simulink model "AariaJoystickR2017a"  (R2017a)
settings: Solver=VariableStepAuto  StartTime=0.0  StopTime=inf  FixedStep=0.1  RelTol=1e-3  EnableMultiTasking=on
model workspace (MATLAB code in the model file):
  | my_a =1;
undefined symbols (not defined in the file or in its folder): AARIAENV, AARIAMAN, AARIASEN, Camera, sensor, Source_TS, X, Y, Z
libraries: sm_lib x723, nesl_utility x640, dspmathops x314, simulink x168, vrlib x2, powerlib_meascontrol x1, aerolibanimutils x1, aerolibutil x1
(part 13 of 26)

== system AariaJoystickR2017a/Tool Sensors/Tool sensor2/placeholder noise2 ==
  Constant : Constant  Value=[1 1 1; 1 1 1; 1 1 1]
  Product : Product
  Uniform Random Number : UniformRandomNumber  Minimum=-0.01  Maximum=0.01  SampleTime=0.1
  noise : Outport
  wires:
  Constant/1 -> Product/1
  Product/1 -> noise/1
  Uniform Random Number/1 -> Product/2

== system AariaJoystickR2017a/Base/BaseVSS/BaseEmpty/IMU Base ==
  Sensor Module1 : Subsystem  mask{nL=nL, nS=1}
      mask prompts: nL "Link Number"; nS "Sensor ID of that link"
      mask DialogControl DescGroupVar Prompt: Virtual IMU
      mask DialogControl DescTextVar Prompt: Measures Connected Body's acceleration and angular velocity in the given point
      mask DialogControl Control2 Prompt: The following numbers defines the corresponding numbers for this sensor to read from the parameters file
  Body Coord : PMIOPort  Port=1  Side=Left
  Reference Coord : PMIOPort  Port=2  Side=Left
  Out1 : Outport
  Out2 : Outport  Port=2
  Out3 : Outport  Port=3
  Out4 : Outport  Port=4
  wires:
  Sensor Module1/3(Out2) -> Out3/1
  Sensor Module1/2(Out4) -> Out2/1
  Sensor Module1/4(Out3) -> Out4/1
  Sensor Module1/1(Out5) -> Out1/1
  connections:
  Sensor Module1/LConn2 -- Reference Coord/RConn1
  Sensor Module1/LConn1 -- Body Coord/RConn1

== system AariaJoystickR2017a/Base/BaseVSS/BaseMotion/IMU Base ==
  Sensor Module1 : Subsystem  mask{nL=nL, nS=1}
      mask prompts: nL "Link Number"; nS "Sensor ID of that link"
      mask DialogControl DescGroupVar Prompt: Virtual IMU
      mask DialogControl DescTextVar Prompt: Measures Connected Body's acceleration and angular velocity in the given point
      mask DialogControl Control2 Prompt: The following numbers defines the corresponding numbers for this sensor to read from the parameters file
  Body Coord : PMIOPort  Port=1  Side=Left
  Reference Coord : PMIOPort  Port=2  Side=Left
  Out1 : Outport
  Out2 : Outport  Port=2
  Out3 : Outport  Port=3
  Out4 : Outport  Port=4
  wires:
  Sensor Module1/3(Out2) -> Out3/1
  Sensor Module1/2(Out4) -> Out2/1
  Sensor Module1/4(Out3) -> Out4/1
  Sensor Module1/1(Out5) -> Out1/1
  connections:
  Sensor Module1/LConn2 -- Reference Coord/RConn1
  Sensor Module1/LConn1 -- Body Coord/RConn1

== system AariaJoystickR2017a/Base/BaseVSS/BaseMotion/x 2motion2 ==
  X : Inport
  Difference : simulink/Discrete/Difference  ICPrevInput=1  InputProcessing=Inherited  OutMin=[]  OutMax=[]  OutDataType=fixdt(1, 16)  OutScaling=2^-10  DoSatur=off
  Difference1 : simulink/Discrete/Difference  ICPrevInput=0  InputProcessing=Inherited  OutMin=[]  OutMax=[]  OutDataType=fixdt(1, 16)  OutScaling=2^-10  DoSatur=off
  Simulink-PS Converter : nesl_utility/Simulink-PS Converter  PhysicalDomain=network_engine_domain  SubClassName=ps_input  LeftPortType=input  RightPortType=output  PseudoPeriodic=off  Frequencies=[]  NoiseDistribution=none  NoiseParameters=[]  Unit=1  AffineConversion=off  FilteringAndDerivatives=provide  SimscapeFilterOrder=1  InputFilterTimeConstant=0.001  UdotUserProvided=2
  Motion for PS : PMIOPort  Port=1  Side=Right
  wires:
  X/1 -> Simulink-PS Converter/1, Difference1/1
  Difference/1 -> Simulink-PS Converter/3
  Difference1/1 -> Difference/1, Simulink-PS Converter/2
  connections:
  Simulink-PS Converter/RConn1 -- Motion for PS/RConn1

== system AariaJoystickR2017a/Base/BaseVSS/BaseMotion/x 2motion3 ==
  X : Inport
  Difference : simulink/Discrete/Difference  ICPrevInput=1  InputProcessing=Inherited  OutMin=[]  OutMax=[]  OutDataType=fixdt(1, 16)  OutScaling=2^-10  DoSatur=off
  Difference1 : simulink/Discrete/Difference  ICPrevInput=0  InputProcessing=Inherited  OutMin=[]  OutMax=[]  OutDataType=fixdt(1, 16)  OutScaling=2^-10  DoSatur=off
  Simulink-PS Converter : nesl_utility/Simulink-PS Converter  PhysicalDomain=network_engine_domain  SubClassName=ps_input  LeftPortType=input  RightPortType=output  PseudoPeriodic=off  Frequencies=[]  NoiseDistribution=none  NoiseParameters=[]  Unit=1  AffineConversion=off  FilteringAndDerivatives=provide  SimscapeFilterOrder=1  InputFilterTimeConstant=0.001  UdotUserProvided=2
  Motion for PS : PMIOPort  Port=1  Side=Right
  wires:
  Difference1/1 -> Simulink-PS Converter/2, Difference/1
  Difference/1 -> Simulink-PS Converter/3
  X/1 -> Difference1/1, Simulink-PS Converter/1
  connections:
  Simulink-PS Converter/RConn1 -- Motion for PS/RConn1

== system AariaJoystickR2017a/Base/BaseVSS/BaseMotion/x 2motion4 ==
  X : Inport
  Difference : simulink/Discrete/Difference  ICPrevInput=1  InputProcessing=Inherited  OutMin=[]  OutMax=[]  OutDataType=fixdt(1, 16)  OutScaling=2^-10  DoSatur=off
  Difference1 : simulink/Discrete/Difference  ICPrevInput=0  InputProcessing=Inherited  OutMin=[]  OutMax=[]  OutDataType=fixdt(1, 16)  OutScaling=2^-10  DoSatur=off
  Simulink-PS Converter : nesl_utility/Simulink-PS Converter  PhysicalDomain=network_engine_domain  SubClassName=ps_input  LeftPortType=input  RightPortType=output  PseudoPeriodic=off  Frequencies=[]  NoiseDistribution=none  NoiseParameters=[]  Unit=1  AffineConversion=off  FilteringAndDerivatives=provide  SimscapeFilterOrder=1  InputFilterTimeConstant=0.001  UdotUserProvided=2
  Motion for PS : PMIOPort  Port=1  Side=Right
  wires:
  X/1 -> Simulink-PS Converter/1, Difference1/1
  Difference/1 -> Simulink-PS Converter/3
  Difference1/1 -> Difference/1, Simulink-PS Converter/2
  connections:
  Simulink-PS Converter/RConn1 -- Motion for PS/RConn1

== system AariaJoystickR2017a/Base/BaseVSS/BaseMotion/x 2motion5 ==
  X : Inport
  Difference : simulink/Discrete/Difference  ICPrevInput=1  InputProcessing=Inherited  OutMin=[]  OutMax=[]  OutDataType=fixdt(1, 16)  OutScaling=2^-10  DoSatur=off
  Difference1 : simulink/Discrete/Difference  ICPrevInput=0  InputProcessing=Inherited  OutMin=[]  OutMax=[]  OutDataType=fixdt(1, 16)  OutScaling=2^-10  DoSatur=off
  Simulink-PS Converter : nesl_utility/Simulink-PS Converter  PhysicalDomain=network_engine_domain  SubClassName=ps_input  LeftPortType=input  RightPortType=output  PseudoPeriodic=off  Frequencies=[]  NoiseDistribution=none  NoiseParameters=[]  Unit=1  AffineConversion=off  FilteringAndDerivatives=provide  SimscapeFilterOrder=1  InputFilterTimeConstant=0.001  UdotUserProvided=2
  Motion for PS : PMIOPort  Port=1  Side=Right
  wires:
  Difference1/1 -> Simulink-PS Converter/2, Difference/1
  Difference/1 -> Simulink-PS Converter/3
  X/1 -> Difference1/1, Simulink-PS Converter/1
  connections:
  Simulink-PS Converter/RConn1 -- Motion for PS/RConn1

== system AariaJoystickR2017a/Base/BaseVSS/BaseMotion/x 2motion6 ==
  X : Inport
  Difference : simulink/Discrete/Difference  ICPrevInput=1  InputProcessing=Inherited  OutMin=[]  OutMax=[]  OutDataType=fixdt(1, 16)  OutScaling=2^-10  DoSatur=off
  Difference1 : simulink/Discrete/Difference  ICPrevInput=0  InputProcessing=Inherited  OutMin=[]  OutMax=[]  OutDataType=fixdt(1, 16)  OutScaling=2^-10  DoSatur=off
  Simulink-PS Converter : nesl_utility/Simulink-PS Converter  PhysicalDomain=network_engine_domain  SubClassName=ps_input  LeftPortType=input  RightPortType=output  PseudoPeriodic=off  Frequencies=[]  NoiseDistribution=none  NoiseParameters=[]  Unit=1  AffineConversion=off  FilteringAndDerivatives=provide  SimscapeFilterOrder=1  InputFilterTimeConstant=0.001  UdotUserProvided=2
  Motion for PS : PMIOPort  Port=1  Side=Right
  wires:
  X/1 -> Simulink-PS Converter/1, Difference1/1
  Difference/1 -> Simulink-PS Converter/3
  Difference1/1 -> Difference/1, Simulink-PS Converter/2
  connections:
  Simulink-PS Converter/RConn1 -- Motion for PS/RConn1

== system AariaJoystickR2017a/Base/BaseVSS/BaseMotion/x 2motion7 ==
  X : Inport
  Difference : simulink/Discrete/Difference  ICPrevInput=1  InputProcessing=Inherited  OutMin=[]  OutMax=[]  OutDataType=fixdt(1, 16)  OutScaling=2^-10  DoSatur=off
  Difference1 : simulink/Discrete/Difference  ICPrevInput=0  InputProcessing=Inherited  OutMin=[]  OutMax=[]  OutDataType=fixdt(1, 16)  OutScaling=2^-10  DoSatur=off
  Simulink-PS Converter : nesl_utility/Simulink-PS Converter  PhysicalDomain=network_engine_domain  SubClassName=ps_input  LeftPortType=input  RightPortType=output  PseudoPeriodic=off  Frequencies=[]  NoiseDistribution=none  NoiseParameters=[]  Unit=1  AffineConversion=off  FilteringAndDerivatives=provide  SimscapeFilterOrder=1  InputFilterTimeConstant=0.001  UdotUserProvided=2
  Motion for PS : PMIOPort  Port=1  Side=Right
  wires:
  Difference1/1 -> Simulink-PS Converter/2, Difference/1
  Difference/1 -> Simulink-PS Converter/3
  X/1 -> Difference1/1, Simulink-PS Converter/1
  connections:
  Simulink-PS Converter/RConn1 -- Motion for PS/RConn1

== system AariaJoystickR2017a/Base/BaseVSS/BaseTorque/IMU Base ==
  Sensor Module1 : Subsystem  mask{nL=nL, nS=1}
      mask prompts: nL "Link Number"; nS "Sensor ID of that link"
      mask DialogControl DescGroupVar Prompt: Virtual IMU
      mask DialogControl DescTextVar Prompt: Measures Connected Body's acceleration and angular velocity in the given point
      mask DialogControl Control2 Prompt: The following numbers defines the corresponding numbers for this sensor to read from the parameters file
  Body Coord : PMIOPort  Port=1  Side=Left
  Reference Coord : PMIOPort  Port=2  Side=Left
  Out1 : Outport
  Out2 : Outport  Port=2
  Out3 : Outport  Port=3
  Out4 : Outport  Port=4
  wires:
  Sensor Module1/3(Out2) -> Out3/1
  Sensor Module1/2(Out4) -> Out2/1
  Sensor Module1/4(Out3) -> Out4/1
  Sensor Module1/1(Out5) -> Out1/1
  connections:
  Sensor Module1/LConn2 -- Reference Coord/RConn1
  Sensor Module1/LConn1 -- Body Coord/RConn1

== system AariaJoystickR2017a/Base/BaseVSS/BaseTorque/x 2motion2 ==
  X : Inport
  Difference : simulink/Discrete/Difference  ICPrevInput=1  InputProcessing=Inherited  OutMin=[]  OutMax=[]  OutDataType=fixdt(1, 16)  OutScaling=2^-10  DoSatur=off
  Difference1 : simulink/Discrete/Difference  ICPrevInput=0  InputProcessing=Inherited  OutMin=[]  OutMax=[]  OutDataType=fixdt(1, 16)  OutScaling=2^-10  DoSatur=off
  Simulink-PS Converter : nesl_utility/Simulink-PS Converter  PhysicalDomain=network_engine_domain  SubClassName=ps_input  LeftPortType=input  RightPortType=output  PseudoPeriodic=off  Frequencies=[]  NoiseDistribution=none  NoiseParameters=[]  Unit=1  AffineConversion=off  FilteringAndDerivatives=provide  SimscapeFilterOrder=1  InputFilterTimeConstant=0.001  UdotUserProvided=2
  Motion for PS : PMIOPort  Port=1  Side=Right
  wires:
  X/1 -> Simulink-PS Converter/1, Difference1/1
  Difference/1 -> Simulink-PS Converter/3
  Difference1/1 -> Difference/1, Simulink-PS Converter/2
  connections:
  Simulink-PS Converter/RConn1 -- Motion for PS/RConn1

== system AariaJoystickR2017a/Base/BaseVSS/BaseTorque/x 2motion3 ==
  X : Inport
  Difference : simulink/Discrete/Difference  ICPrevInput=1  InputProcessing=Inherited  OutMin=[]  OutMax=[]  OutDataType=fixdt(1, 16)  OutScaling=2^-10  DoSatur=off
  Difference1 : simulink/Discrete/Difference  ICPrevInput=0  InputProcessing=Inherited  OutMin=[]  OutMax=[]  OutDataType=fixdt(1, 16)  OutScaling=2^-10  DoSatur=off
  Simulink-PS Converter : nesl_utility/Simulink-PS Converter  PhysicalDomain=network_engine_domain  SubClassName=ps_input  LeftPortType=input  RightPortType=output  PseudoPeriodic=off  Frequencies=[]  NoiseDistribution=none  NoiseParameters=[]  Unit=1  AffineConversion=off  FilteringAndDerivatives=provide  SimscapeFilterOrder=1  InputFilterTimeConstant=0.001  UdotUserProvided=2
  Motion for PS : PMIOPort  Port=1  Side=Right
  wires:
  Difference1/1 -> Simulink-PS Converter/2, Difference/1
  Difference/1 -> Simulink-PS Converter/3
  X/1 -> Difference1/1, Simulink-PS Converter/1
  connections:
  Simulink-PS Converter/RConn1 -- Motion for PS/RConn1

== system AariaJoystickR2017a/Base/BaseVSS/BaseTorque/x 2motion4 ==
  X : Inport
  Difference : simulink/Discrete/Difference  ICPrevInput=1  InputProcessing=Inherited  OutMin=[]  OutMax=[]  OutDataType=fixdt(1, 16)  OutScaling=2^-10  DoSatur=off
  Difference1 : simulink/Discrete/Difference  ICPrevInput=0  InputProcessing=Inherited  OutMin=[]  OutMax=[]  OutDataType=fixdt(1, 16)  OutScaling=2^-10  DoSatur=off
  Simulink-PS Converter : nesl_utility/Simulink-PS Converter  PhysicalDomain=network_engine_domain  SubClassName=ps_input  LeftPortType=input  RightPortType=output  PseudoPeriodic=off  Frequencies=[]  NoiseDistribution=none  NoiseParameters=[]  Unit=1  AffineConversion=off  FilteringAndDerivatives=provide  SimscapeFilterOrder=1  InputFilterTimeConstant=0.001  UdotUserProvided=2
  Motion for PS : PMIOPort  Port=1  Side=Right
  wires:
  X/1 -> Simulink-PS Converter/1, Difference1/1
  Difference/1 -> Simulink-PS Converter/3
  Difference1/1 -> Difference/1, Simulink-PS Converter/2
  connections:
  Simulink-PS Converter/RConn1 -- Motion for PS/RConn1

== system AariaJoystickR2017a/Base/BaseVSS/BaseTorque/x 2motion5 ==
  X : Inport
  Difference : simulink/Discrete/Difference  ICPrevInput=1  InputProcessing=Inherited  OutMin=[]  OutMax=[]  OutDataType=fixdt(1, 16)  OutScaling=2^-10  DoSatur=off
  Difference1 : simulink/Discrete/Difference  ICPrevInput=0  InputProcessing=Inherited  OutMin=[]  OutMax=[]  OutDataType=fixdt(1, 16)  OutScaling=2^-10  DoSatur=off
  Simulink-PS Converter : nesl_utility/Simulink-PS Converter  PhysicalDomain=network_engine_domain  SubClassName=ps_input  LeftPortType=input  RightPortType=output  PseudoPeriodic=off  Frequencies=[]  NoiseDistribution=none  NoiseParameters=[]  Unit=1  AffineConversion=off  FilteringAndDerivatives=provide  SimscapeFilterOrder=1  InputFilterTimeConstant=0.001  UdotUserProvided=2
  Motion for PS : PMIOPort  Port=1  Side=Right
  wires:
  Difference1/1 -> Simulink-PS Converter/2, Difference/1
  Difference/1 -> Simulink-PS Converter/3
  X/1 -> Difference1/1, Simulink-PS Converter/1
  connections:
  Simulink-PS Converter/RConn1 -- Motion for PS/RConn1

== system AariaJoystickR2017a/Base/BaseVSS/BaseTorque/x 2motion6 ==
  X : Inport
  Difference : simulink/Discrete/Difference  ICPrevInput=1  InputProcessing=Inherited  OutMin=[]  OutMax=[]  OutDataType=fixdt(1, 16)  OutScaling=2^-10  DoSatur=off
  Difference1 : simulink/Discrete/Difference  ICPrevInput=0  InputProcessing=Inherited  OutMin=[]  OutMax=[]  OutDataType=fixdt(1, 16)  OutScaling=2^-10  DoSatur=off
  Simulink-PS Converter : nesl_utility/Simulink-PS Converter  PhysicalDomain=network_engine_domain  SubClassName=ps_input  LeftPortType=input  RightPortType=output  PseudoPeriodic=off  Frequencies=[]  NoiseDistribution=none  NoiseParameters=[]  Unit=1  AffineConversion=off  FilteringAndDerivatives=provide  SimscapeFilterOrder=1  InputFilterTimeConstant=0.001  UdotUserProvided=2
  Motion for PS : PMIOPort  Port=1  Side=Right
  wires:
  X/1 -> Simulink-PS Converter/1, Difference1/1
  Difference/1 -> Simulink-PS Converter/3
  Difference1/1 -> Difference/1, Simulink-PS Converter/2
  connections:
  Simulink-PS Converter/RConn1 -- Motion for PS/RConn1

== system AariaJoystickR2017a/Base/BaseVSS/BaseTorque/x 2motion7 ==
  X : Inport
  Difference : simulink/Discrete/Difference  ICPrevInput=1  InputProcessing=Inherited  OutMin=[]  OutMax=[]  OutDataType=fixdt(1, 16)  OutScaling=2^-10  DoSatur=off
  Difference1 : simulink/Discrete/Difference  ICPrevInput=0  InputProcessing=Inherited  OutMin=[]  OutMax=[]  OutDataType=fixdt(1, 16)  OutScaling=2^-10  DoSatur=off
  Simulink-PS Converter : nesl_utility/Simulink-PS Converter  PhysicalDomain=network_engine_domain  SubClassName=ps_input  LeftPortType=input  RightPortType=output  PseudoPeriodic=off  Frequencies=[]  NoiseDistribution=none  NoiseParameters=[]  Unit=1  AffineConversion=off  FilteringAndDerivatives=provide  SimscapeFilterOrder=1  InputFilterTimeConstant=0.001  UdotUserProvided=2
  Motion for PS : PMIOPort  Port=1  Side=Right
  wires:
  Difference1/1 -> Simulink-PS Converter/2, Difference/1
  Difference/1 -> Simulink-PS Converter/3
  X/1 -> Difference1/1, Simulink-PS Converter/1
  connections:
  Simulink-PS Converter/RConn1 -- Motion for PS/RConn1

== system AariaJoystickR2017a/Joint1/JointVSS/PrismaticMotion/IMU Sensors ==
  Sensor Module1 : Subsystem  mask{nL=nL, nS=1}
      mask prompts: nL "Link Number"; nS "Sensor ID of that link"
      mask DialogControl DescGroupVar Prompt: Virtual IMU
      mask DialogControl DescTextVar Prompt: Measures Connected Body's acceleration and angular velocity in the given point
      mask DialogControl Control2 Prompt: The following numbers defines the corresponding numbers for this sensor to read from the parameters file
  Sensor Module2 : Subsystem  mask{nL=nL, nS=2}
      mask prompts: nL "Link Number"; nS "Sensor ID of that link"
      mask DialogControl DescGroupVar Prompt: Virtual IMU
      mask DialogControl DescTextVar Prompt: Measures Connected Body's acceleration and angular velocity in the given point
      mask DialogControl Control2 Prompt: The following numbers defines the corresponding numbers for this sensor to read from the parameters file
  Terminator{,1..3} (4 alike) : Terminator
  Body Coord : PMIOPort  Port=1  Side=Left
  Reference Coord : PMIOPort  Port=2  Side=Left
  Out1 : Outport
  Out2 : Outport  Port=2
  Out5 : Outport  Port=3
  Out6 : Outport  Port=4
  wires:
  Sensor Module2/3(Out2) -> Terminator2/1
  Sensor Module2/1(Out5) -> Out5/1
  Sensor Module2/4(Out3) -> Terminator3/1
  Sensor Module2/2(Out4) -> Out6/1
  Sensor Module1/1(Out5) -> Out1/1
  Sensor Module1/4(Out3) -> Terminator1/1
  Sensor Module1/2(Out4) -> Out2/1
  Sensor Module1/3(Out2) -> Terminator/1
  connections:
  Sensor Module1/LConn1 -- Body Coord/RConn1 -- Sensor Module2/LConn1
  Sensor Module1/LConn2 -- Reference Coord/RConn1 -- Sensor Module2/LConn2

== system AariaJoystickR2017a/Joint1/JointVSS/PrismaticMotion/x 2motion ==
  X : Inport
  Difference : simulink/Discrete/Difference  ICPrevInput=1  InputProcessing=Inherited  OutMin=[]  OutMax=[]  OutDataType=fixdt(1, 16)  OutScaling=2^-10  DoSatur=off
  Difference1 : simulink/Discrete/Difference  ICPrevInput=0  InputProcessing=Inherited  OutMin=[]  OutMax=[]  OutDataType=fixdt(1, 16)  OutScaling=2^-10  DoSatur=off
  Simulink-PS Converter : nesl_utility/Simulink-PS Converter  PhysicalDomain=network_engine_domain  SubClassName=ps_input  LeftPortType=input  RightPortType=output  PseudoPeriodic=off  Frequencies=[]  NoiseDistribution=none  NoiseParameters=[]  Unit=1  AffineConversion=off  FilteringAndDerivatives=provide  SimscapeFilterOrder=1  InputFilterTimeConstant=0.001  UdotUserProvided=2
  Motion for PS : PMIOPort  Port=1  Side=Right
  wires:
  X/1 -> Simulink-PS Converter/1, Difference1/1
  Difference/1 -> Simulink-PS Converter/3
  Difference1/1 -> Difference/1, Simulink-PS Converter/2
  connections:
  Simulink-PS Converter/RConn1 -- Motion for PS/RConn1

== system AariaJoystickR2017a/Joint1/JointVSS/PrismaticTorque/IMU Sensors ==
  Sensor Module1 : Subsystem  mask{nL=nL, nS=1}
      mask prompts: nL "Link Number"; nS "Sensor ID of that link"
      mask DialogControl DescGroupVar Prompt: Virtual IMU
      mask DialogControl DescTextVar Prompt: Measures Connected Body's acceleration and angular velocity in the given point
      mask DialogControl Control2 Prompt: The following numbers defines the corresponding numbers for this sensor to read from the parameters file
  Sensor Module2 : Subsystem  mask{nL=nL, nS=2}
      mask prompts: nL "Link Number"; nS "Sensor ID of that link"
      mask DialogControl DescGroupVar Prompt: Virtual IMU
      mask DialogControl DescTextVar Prompt: Measures Connected Body's acceleration and angular velocity in the given point
      mask DialogControl Control2 Prompt: The following numbers defines the corresponding numbers for this sensor to read from the parameters file
  Terminator{,1..3} (4 alike) : Terminator
  Body Coord : PMIOPort  Port=1  Side=Left
  Reference Coord : PMIOPort  Port=2  Side=Left
  Out1 : Outport
  Out2 : Outport  Port=2
  Out5 : Outport  Port=3
  Out6 : Outport  Port=4
  wires:
  Sensor Module2/3(Out2) -> Terminator2/1
  Sensor Module2/1(Out5) -> Out5/1
  Sensor Module2/4(Out3) -> Terminator3/1
  Sensor Module2/2(Out4) -> Out6/1
  Sensor Module1/1(Out5) -> Out1/1
  Sensor Module1/4(Out3) -> Terminator1/1
  Sensor Module1/2(Out4) -> Out2/1
  Sensor Module1/3(Out2) -> Terminator/1
  connections:
  Sensor Module1/LConn1 -- Body Coord/RConn1 -- Sensor Module2/LConn1
  Sensor Module1/LConn2 -- Reference Coord/RConn1 -- Sensor Module2/LConn2

== system AariaJoystickR2017a/Joint1/JointVSS/RevoluteMotion/IMU Sensors ==
  Sensor Module1 : Subsystem  mask{nL=nL, nS=1}
      mask prompts: nL "Link Number"; nS "Sensor ID of that link"
      mask DialogControl DescGroupVar Prompt: Virtual IMU
      mask DialogControl DescTextVar Prompt: Measures Connected Body's acceleration and angular velocity in the given point
      mask DialogControl Control2 Prompt: The following numbers defines the corresponding numbers for this sensor to read from the parameters file
  Sensor Module2 : Subsystem  mask{nL=nL, nS=2}
      mask prompts: nL "Link Number"; nS "Sensor ID of that link"
      mask DialogControl DescGroupVar Prompt: Virtual IMU
      mask DialogControl DescTextVar Prompt: Measures Connected Body's acceleration and angular velocity in the given point
      mask DialogControl Control2 Prompt: The following numbers defines the corresponding numbers for this sensor to read from the parameters file
  Terminator{,1..3} (4 alike) : Terminator
  Body Coord : PMIOPort  Port=1  Side=Left
  Reference Coord : PMIOPort  Port=2  Side=Left
  Out1 : Outport
  Out2 : Outport  Port=2
  Out5 : Outport  Port=3
  Out6 : Outport  Port=4
  wires:
  Sensor Module2/3(Out2) -> Terminator2/1
  Sensor Module2/1(Out5) -> Out5/1
  Sensor Module2/4(Out3) -> Terminator3/1
  Sensor Module2/2(Out4) -> Out6/1
  Sensor Module1/1(Out5) -> Out1/1
  Sensor Module1/4(Out3) -> Terminator1/1
  Sensor Module1/2(Out4) -> Out2/1
  Sensor Module1/3(Out2) -> Terminator/1
  connections:
  Sensor Module1/LConn1 -- Body Coord/RConn1 -- Sensor Module2/LConn1
  Sensor Module1/LConn2 -- Reference Coord/RConn1 -- Sensor Module2/LConn2

== system AariaJoystickR2017a/Joint1/JointVSS/RevoluteMotion/x 2motion ==
  X : Inport
  Difference : simulink/Discrete/Difference  ICPrevInput=1  InputProcessing=Inherited  OutMin=[]  OutMax=[]  OutDataType=fixdt(1, 16)  OutScaling=2^-10  DoSatur=off
  Difference1 : simulink/Discrete/Difference  ICPrevInput=0  InputProcessing=Inherited  OutMin=[]  OutMax=[]  OutDataType=fixdt(1, 16)  OutScaling=2^-10  DoSatur=off
  Simulink-PS Converter : nesl_utility/Simulink-PS Converter  PhysicalDomain=network_engine_domain  SubClassName=ps_input  LeftPortType=input  RightPortType=output  PseudoPeriodic=off  Frequencies=[]  NoiseDistribution=none  NoiseParameters=[]  Unit=1  AffineConversion=off  FilteringAndDerivatives=provide  SimscapeFilterOrder=1  InputFilterTimeConstant=0.001  UdotUserProvided=2
  Motion for PS : PMIOPort  Port=1  Side=Right
  wires:
  Difference1/1 -> Simulink-PS Converter/2, Difference/1
  Difference/1 -> Simulink-PS Converter/3
  X/1 -> Difference1/1, Simulink-PS Converter/1
  connections:
  Simulink-PS Converter/RConn1 -- Motion for PS/RConn1

== system AariaJoystickR2017a/Joint1/JointVSS/RevoluteTorque/IMU Sensors ==
  Sensor Module1 : Subsystem  mask{nL=nL, nS=1}
      mask prompts: nL "Link Number"; nS "Sensor ID of that link"
      mask DialogControl DescGroupVar Prompt: Virtual IMU
      mask DialogControl DescTextVar Prompt: Measures Connected Body's acceleration and angular velocity in the given point
      mask DialogControl Control2 Prompt: The following numbers defines the corresponding numbers for this sensor to read from the parameters file
  Sensor Module2 : Subsystem  mask{nL=nL, nS=2}
      mask prompts: nL "Link Number"; nS "Sensor ID of that link"
      mask DialogControl DescGroupVar Prompt: Virtual IMU
      mask DialogControl DescTextVar Prompt: Measures Connected Body's acceleration and angular velocity in the given point
      mask DialogControl Control2 Prompt: The following numbers defines the corresponding numbers for this sensor to read from the parameters file
  Terminator{,1..3} (4 alike) : Terminator
  Body Coord : PMIOPort  Port=1  Side=Left
  Reference Coord : PMIOPort  Port=2  Side=Left
  Out1 : Outport
  Out2 : Outport  Port=2
  Out5 : Outport  Port=3
  Out6 : Outport  Port=4
  wires:
  Sensor Module2/3(Out2) -> Terminator2/1
  Sensor Module2/1(Out5) -> Out5/1
  Sensor Module2/4(Out3) -> Terminator3/1
  Sensor Module2/2(Out4) -> Out6/1
  Sensor Module1/1(Out5) -> Out1/1
  Sensor Module1/4(Out3) -> Terminator1/1
  Sensor Module1/2(Out4) -> Out2/1
  Sensor Module1/3(Out2) -> Terminator/1
  connections:
  Sensor Module1/LConn1 -- Body Coord/RConn1 -- Sensor Module2/LConn1
  Sensor Module1/LConn2 -- Reference Coord/RConn1 -- Sensor Module2/LConn2

== system AariaJoystickR2017a/Joint2/JointVSS/PrismaticMotion/IMU Sensors ==
  Sensor Module1 : Subsystem  mask{nL=nL, nS=1}
      mask prompts: nL "Link Number"; nS "Sensor ID of that link"
      mask DialogControl DescGroupVar Prompt: Virtual IMU
      mask DialogControl DescTextVar Prompt: Measures Connected Body's acceleration and angular velocity in the given point
      mask DialogControl Control2 Prompt: The following numbers defines the corresponding numbers for this sensor to read from the parameters file
  Sensor Module2 : Subsystem  mask{nL=nL, nS=2}
      mask prompts: nL "Link Number"; nS "Sensor ID of that link"
      mask DialogControl DescGroupVar Prompt: Virtual IMU
      mask DialogControl DescTextVar Prompt: Measures Connected Body's acceleration and angular velocity in the given point
      mask DialogControl Control2 Prompt: The following numbers defines the corresponding numbers for this sensor to read from the parameters file
  Terminator{,1..3} (4 alike) : Terminator
  Body Coord : PMIOPort  Port=1  Side=Left
  Reference Coord : PMIOPort  Port=2  Side=Left
  Out1 : Outport
  Out2 : Outport  Port=2
  Out5 : Outport  Port=3
  Out6 : Outport  Port=4
  wires:
  Sensor Module1/3(Out2) -> Terminator/1
  Sensor Module1/2(Out4) -> Out2/1
  Sensor Module1/4(Out3) -> Terminator1/1
  Sensor Module1/1(Out5) -> Out1/1
  Sensor Module2/2(Out4) -> Out6/1
  Sensor Module2/4(Out3) -> Terminator3/1
  Sensor Module2/1(Out5) -> Out5/1
  Sensor Module2/3(Out2) -> Terminator2/1
  connections:
  Sensor Module2/LConn2 -- Reference Coord/RConn1 -- Sensor Module1/LConn2
  Sensor Module2/LConn1 -- Body Coord/RConn1 -- Sensor Module1/LConn1

== system AariaJoystickR2017a/Joint2/JointVSS/PrismaticMotion/x 2motion ==
  X : Inport
  Difference : simulink/Discrete/Difference  ICPrevInput=1  InputProcessing=Inherited  OutMin=[]  OutMax=[]  OutDataType=fixdt(1, 16)  OutScaling=2^-10  DoSatur=off
  Difference1 : simulink/Discrete/Difference  ICPrevInput=0  InputProcessing=Inherited  OutMin=[]  OutMax=[]  OutDataType=fixdt(1, 16)  OutScaling=2^-10  DoSatur=off
  Simulink-PS Converter : nesl_utility/Simulink-PS Converter  PhysicalDomain=network_engine_domain  SubClassName=ps_input  LeftPortType=input  RightPortType=output  PseudoPeriodic=off  Frequencies=[]  NoiseDistribution=none  NoiseParameters=[]  Unit=1  AffineConversion=off  FilteringAndDerivatives=provide  SimscapeFilterOrder=1  InputFilterTimeConstant=0.001  UdotUserProvided=2
  Motion for PS : PMIOPort  Port=1  Side=Right
  wires:
  Difference1/1 -> Simulink-PS Converter/2, Difference/1
  Difference/1 -> Simulink-PS Converter/3
  X/1 -> Difference1/1, Simulink-PS Converter/1
  connections:
  Simulink-PS Converter/RConn1 -- Motion for PS/RConn1

== system AariaJoystickR2017a/Joint2/JointVSS/PrismaticTorque/IMU Sensors ==
  Sensor Module1 : Subsystem  mask{nL=nL, nS=1}
      mask prompts: nL "Link Number"; nS "Sensor ID of that link"
      mask DialogControl DescGroupVar Prompt: Virtual IMU
      mask DialogControl DescTextVar Prompt: Measures Connected Body's acceleration and angular velocity in the given point
      mask DialogControl Control2 Prompt: The following numbers defines the corresponding numbers for this sensor to read from the parameters file
  Sensor Module2 : Subsystem  mask{nL=nL, nS=2}
      mask prompts: nL "Link Number"; nS "Sensor ID of that link"
      mask DialogControl DescGroupVar Prompt: Virtual IMU
      mask DialogControl DescTextVar Prompt: Measures Connected Body's acceleration and angular velocity in the given point
      mask DialogControl Control2 Prompt: The following numbers defines the corresponding numbers for this sensor to read from the parameters file
  Terminator{,1..3} (4 alike) : Terminator
  Body Coord : PMIOPort  Port=1  Side=Left
  Reference Coord : PMIOPort  Port=2  Side=Left
  Out1 : Outport
  Out2 : Outport  Port=2
  Out5 : Outport  Port=3
  Out6 : Outport  Port=4
  wires:
  Sensor Module1/3(Out2) -> Terminator/1
  Sensor Module1/2(Out4) -> Out2/1
  Sensor Module1/4(Out3) -> Terminator1/1
  Sensor Module1/1(Out5) -> Out1/1
  Sensor Module2/2(Out4) -> Out6/1
  Sensor Module2/4(Out3) -> Terminator3/1
  Sensor Module2/1(Out5) -> Out5/1
  Sensor Module2/3(Out2) -> Terminator2/1
  connections:
  Sensor Module2/LConn2 -- Reference Coord/RConn1 -- Sensor Module1/LConn2
  Sensor Module2/LConn1 -- Body Coord/RConn1 -- Sensor Module1/LConn1

== system AariaJoystickR2017a/Joint2/JointVSS/RevoluteMotion/IMU Sensors ==
  Sensor Module1 : Subsystem  mask{nL=nL, nS=1}
      mask prompts: nL "Link Number"; nS "Sensor ID of that link"
      mask DialogControl DescGroupVar Prompt: Virtual IMU
      mask DialogControl DescTextVar Prompt: Measures Connected Body's acceleration and angular velocity in the given point
      mask DialogControl Control2 Prompt: The following numbers defines the corresponding numbers for this sensor to read from the parameters file
  Sensor Module2 : Subsystem  mask{nL=nL, nS=2}
      mask prompts: nL "Link Number"; nS "Sensor ID of that link"
      mask DialogControl DescGroupVar Prompt: Virtual IMU
      mask DialogControl DescTextVar Prompt: Measures Connected Body's acceleration and angular velocity in the given point
      mask DialogControl Control2 Prompt: The following numbers defines the corresponding numbers for this sensor to read from the parameters file
  Terminator{,1..3} (4 alike) : Terminator
  Body Coord : PMIOPort  Port=1  Side=Left
  Reference Coord : PMIOPort  Port=2  Side=Left
  Out1 : Outport
  Out2 : Outport  Port=2
  Out5 : Outport  Port=3
  Out6 : Outport  Port=4
  wires:
  Sensor Module1/3(Out2) -> Terminator/1
  Sensor Module1/2(Out4) -> Out2/1
  Sensor Module1/4(Out3) -> Terminator1/1
  Sensor Module1/1(Out5) -> Out1/1
  Sensor Module2/2(Out4) -> Out6/1
  Sensor Module2/4(Out3) -> Terminator3/1
  Sensor Module2/1(Out5) -> Out5/1
  Sensor Module2/3(Out2) -> Terminator2/1
  connections:
  Sensor Module2/LConn2 -- Reference Coord/RConn1 -- Sensor Module1/LConn2
  Sensor Module2/LConn1 -- Body Coord/RConn1 -- Sensor Module1/LConn1

== system AariaJoystickR2017a/Joint2/JointVSS/RevoluteMotion/x 2motion ==
  X : Inport
  Difference : simulink/Discrete/Difference  ICPrevInput=1  InputProcessing=Inherited  OutMin=[]  OutMax=[]  OutDataType=fixdt(1, 16)  OutScaling=2^-10  DoSatur=off
  Difference1 : simulink/Discrete/Difference  ICPrevInput=0  InputProcessing=Inherited  OutMin=[]  OutMax=[]  OutDataType=fixdt(1, 16)  OutScaling=2^-10  DoSatur=off
  Simulink-PS Converter : nesl_utility/Simulink-PS Converter  PhysicalDomain=network_engine_domain  SubClassName=ps_input  LeftPortType=input  RightPortType=output  PseudoPeriodic=off  Frequencies=[]  NoiseDistribution=none  NoiseParameters=[]  Unit=1  AffineConversion=off  FilteringAndDerivatives=provide  SimscapeFilterOrder=1  InputFilterTimeConstant=0.001  UdotUserProvided=2
  Motion for PS : PMIOPort  Port=1  Side=Right
  wires:
  X/1 -> Simulink-PS Converter/1, Difference1/1
  Difference/1 -> Simulink-PS Converter/3
  Difference1/1 -> Difference/1, Simulink-PS Converter/2
  connections:
  Simulink-PS Converter/RConn1 -- Motion for PS/RConn1

== system AariaJoystickR2017a/Joint2/JointVSS/RevoluteTorque/IMU Sensors ==
  Sensor Module1 : Subsystem  mask{nL=nL, nS=1}
      mask prompts: nL "Link Number"; nS "Sensor ID of that link"
      mask DialogControl DescGroupVar Prompt: Virtual IMU
      mask DialogControl DescTextVar Prompt: Measures Connected Body's acceleration and angular velocity in the given point
      mask DialogControl Control2 Prompt: The following numbers defines the corresponding numbers for this sensor to read from the parameters file
  Sensor Module2 : Subsystem  mask{nL=nL, nS=2}
      mask prompts: nL "Link Number"; nS "Sensor ID of that link"
      mask DialogControl DescGroupVar Prompt: Virtual IMU
      mask DialogControl DescTextVar Prompt: Measures Connected Body's acceleration and angular velocity in the given point
      mask DialogControl Control2 Prompt: The following numbers defines the corresponding numbers for this sensor to read from the parameters file
  Terminator{,1..3} (4 alike) : Terminator
  Body Coord : PMIOPort  Port=1  Side=Left
  Reference Coord : PMIOPort  Port=2  Side=Left
  Out1 : Outport
  Out2 : Outport  Port=2
  Out5 : Outport  Port=3
  Out6 : Outport  Port=4
  wires:
  Sensor Module1/3(Out2) -> Terminator/1
  Sensor Module1/2(Out4) -> Out2/1
  Sensor Module1/4(Out3) -> Terminator1/1
  Sensor Module1/1(Out5) -> Out1/1
  Sensor Module2/2(Out4) -> Out6/1
  Sensor Module2/4(Out3) -> Terminator3/1
  Sensor Module2/1(Out5) -> Out5/1
  Sensor Module2/3(Out2) -> Terminator2/1
  connections:
  Sensor Module2/LConn2 -- Reference Coord/RConn1 -- Sensor Module1/LConn2
  Sensor Module2/LConn1 -- Body Coord/RConn1 -- Sensor Module1/LConn1

== system AariaJoystickR2017a/Joint3/JointVSS/PrismaticMotion/IMU Sensors ==
  Sensor Module1 : Subsystem  mask{nL=nL, nS=1}
      mask prompts: nL "Link Number"; nS "Sensor ID of that link"
      mask DialogControl DescGroupVar Prompt: Virtual IMU
      mask DialogControl DescTextVar Prompt: Measures Connected Body's acceleration and angular velocity in the given point
      mask DialogControl Control2 Prompt: The following numbers defines the corresponding numbers for this sensor to read from the parameters file
  Sensor Module2 : Subsystem  mask{nL=nL, nS=2}
      mask prompts: nL "Link Number"; nS "Sensor ID of that link"
      mask DialogControl DescGroupVar Prompt: Virtual IMU
      mask DialogControl DescTextVar Prompt: Measures Connected Body's acceleration and angular velocity in the given point
      mask DialogControl Control2 Prompt: The following numbers defines the corresponding numbers for this sensor to read from the parameters file
  Terminator{,1..3} (4 alike) : Terminator
  Body Coord : PMIOPort  Port=1  Side=Left
  Reference Coord : PMIOPort  Port=2  Side=Left
  Out1 : Outport
  Out2 : Outport  Port=2
  Out5 : Outport  Port=3
  Out6 : Outport  Port=4
  wires:
  Sensor Module2/3(Out2) -> Terminator2/1
  Sensor Module2/1(Out5) -> Out5/1
  Sensor Module2/4(Out3) -> Terminator3/1
  Sensor Module2/2(Out4) -> Out6/1
  Sensor Module1/1(Out5) -> Out1/1
  Sensor Module1/4(Out3) -> Terminator1/1
  Sensor Module1/2(Out4) -> Out2/1
  Sensor Module1/3(Out2) -> Terminator/1
  connections:
  Sensor Module1/LConn1 -- Body Coord/RConn1 -- Sensor Module2/LConn1
  Sensor Module1/LConn2 -- Reference Coord/RConn1 -- Sensor Module2/LConn2

== system AariaJoystickR2017a/Joint3/JointVSS/PrismaticMotion/x 2motion ==
  X : Inport
  Difference : simulink/Discrete/Difference  ICPrevInput=1  InputProcessing=Inherited  OutMin=[]  OutMax=[]  OutDataType=fixdt(1, 16)  OutScaling=2^-10  DoSatur=off
  Difference1 : simulink/Discrete/Difference  ICPrevInput=0  InputProcessing=Inherited  OutMin=[]  OutMax=[]  OutDataType=fixdt(1, 16)  OutScaling=2^-10  DoSatur=off
  Simulink-PS Converter : nesl_utility/Simulink-PS Converter  PhysicalDomain=network_engine_domain  SubClassName=ps_input  LeftPortType=input  RightPortType=output  PseudoPeriodic=off  Frequencies=[]  NoiseDistribution=none  NoiseParameters=[]  Unit=1  AffineConversion=off  FilteringAndDerivatives=provide  SimscapeFilterOrder=1  InputFilterTimeConstant=0.001  UdotUserProvided=2
  Motion for PS : PMIOPort  Port=1  Side=Right
  wires:
  X/1 -> Simulink-PS Converter/1, Difference1/1
  Difference/1 -> Simulink-PS Converter/3
  Difference1/1 -> Difference/1, Simulink-PS Converter/2
  connections:
  Simulink-PS Converter/RConn1 -- Motion for PS/RConn1

== system AariaJoystickR2017a/Joint3/JointVSS/PrismaticTorque/IMU Sensors ==
  Sensor Module1 : Subsystem  mask{nL=nL, nS=1}
      mask prompts: nL "Link Number"; nS "Sensor ID of that link"
      mask DialogControl DescGroupVar Prompt: Virtual IMU
      mask DialogControl DescTextVar Prompt: Measures Connected Body's acceleration and angular velocity in the given point
      mask DialogControl Control2 Prompt: The following numbers defines the corresponding numbers for this sensor to read from the parameters file
  Sensor Module2 : Subsystem  mask{nL=nL, nS=2}
      mask prompts: nL "Link Number"; nS "Sensor ID of that link"
      mask DialogControl DescGroupVar Prompt: Virtual IMU
      mask DialogControl DescTextVar Prompt: Measures Connected Body's acceleration and angular velocity in the given point
      mask DialogControl Control2 Prompt: The following numbers defines the corresponding numbers for this sensor to read from the parameters file
  Terminator{,1..3} (4 alike) : Terminator
  Body Coord : PMIOPort  Port=1  Side=Left
  Reference Coord : PMIOPort  Port=2  Side=Left
  Out1 : Outport
  Out2 : Outport  Port=2
  Out5 : Outport  Port=3
  Out6 : Outport  Port=4
  wires:
  Sensor Module2/3(Out2) -> Terminator2/1
  Sensor Module2/1(Out5) -> Out5/1
  Sensor Module2/4(Out3) -> Terminator3/1
  Sensor Module2/2(Out4) -> Out6/1
  Sensor Module1/1(Out5) -> Out1/1
  Sensor Module1/4(Out3) -> Terminator1/1
  Sensor Module1/2(Out4) -> Out2/1
  Sensor Module1/3(Out2) -> Terminator/1
  connections:
  Sensor Module1/LConn1 -- Body Coord/RConn1 -- Sensor Module2/LConn1
  Sensor Module1/LConn2 -- Reference Coord/RConn1 -- Sensor Module2/LConn2

== system AariaJoystickR2017a/Joint3/JointVSS/RevoluteMotion/IMU Sensors ==
  Sensor Module1 : Subsystem  mask{nL=nL, nS=1}
      mask prompts: nL "Link Number"; nS "Sensor ID of that link"
      mask DialogControl DescGroupVar Prompt: Virtual IMU
      mask DialogControl DescTextVar Prompt: Measures Connected Body's acceleration and angular velocity in the given point
      mask DialogControl Control2 Prompt: The following numbers defines the corresponding numbers for this sensor to read from the parameters file
  Sensor Module2 : Subsystem  mask{nL=nL, nS=2}
      mask prompts: nL "Link Number"; nS "Sensor ID of that link"
      mask DialogControl DescGroupVar Prompt: Virtual IMU
      mask DialogControl DescTextVar Prompt: Measures Connected Body's acceleration and angular velocity in the given point
      mask DialogControl Control2 Prompt: The following numbers defines the corresponding numbers for this sensor to read from the parameters file
  Terminator{,1..3} (4 alike) : Terminator
  Body Coord : PMIOPort  Port=1  Side=Left
  Reference Coord : PMIOPort  Port=2  Side=Left
  Out1 : Outport
  Out2 : Outport  Port=2
  Out5 : Outport  Port=3
  Out6 : Outport  Port=4
  wires:
  Sensor Module2/3(Out2) -> Terminator2/1
  Sensor Module2/1(Out5) -> Out5/1
  Sensor Module2/4(Out3) -> Terminator3/1
  Sensor Module2/2(Out4) -> Out6/1
  Sensor Module1/1(Out5) -> Out1/1
  Sensor Module1/4(Out3) -> Terminator1/1
  Sensor Module1/2(Out4) -> Out2/1
  Sensor Module1/3(Out2) -> Terminator/1
  connections:
  Sensor Module1/LConn1 -- Body Coord/RConn1 -- Sensor Module2/LConn1
  Sensor Module1/LConn2 -- Reference Coord/RConn1 -- Sensor Module2/LConn2

== system AariaJoystickR2017a/Joint3/JointVSS/RevoluteMotion/x 2motion ==
  X : Inport
  Difference : simulink/Discrete/Difference  ICPrevInput=1  InputProcessing=Inherited  OutMin=[]  OutMax=[]  OutDataType=fixdt(1, 16)  OutScaling=2^-10  DoSatur=off
  Difference1 : simulink/Discrete/Difference  ICPrevInput=0  InputProcessing=Inherited  OutMin=[]  OutMax=[]  OutDataType=fixdt(1, 16)  OutScaling=2^-10  DoSatur=off
  Simulink-PS Converter : nesl_utility/Simulink-PS Converter  PhysicalDomain=network_engine_domain  SubClassName=ps_input  LeftPortType=input  RightPortType=output  PseudoPeriodic=off  Frequencies=[]  NoiseDistribution=none  NoiseParameters=[]  Unit=1  AffineConversion=off  FilteringAndDerivatives=provide  SimscapeFilterOrder=1  InputFilterTimeConstant=0.001  UdotUserProvided=2
  Motion for PS : PMIOPort  Port=1  Side=Right
  wires:
  Difference1/1 -> Simulink-PS Converter/2, Difference/1
  Difference/1 -> Simulink-PS Converter/3
  X/1 -> Difference1/1, Simulink-PS Converter/1
  connections:
  Simulink-PS Converter/RConn1 -- Motion for PS/RConn1

== system AariaJoystickR2017a/Joint3/JointVSS/RevoluteTorque/IMU Sensors ==
  Sensor Module1 : Subsystem  mask{nL=nL, nS=1}
      mask prompts: nL "Link Number"; nS "Sensor ID of that link"
      mask DialogControl DescGroupVar Prompt: Virtual IMU
      mask DialogControl DescTextVar Prompt: Measures Connected Body's acceleration and angular velocity in the given point
      mask DialogControl Control2 Prompt: The following numbers defines the corresponding numbers for this sensor to read from the parameters file
  Sensor Module2 : Subsystem  mask{nL=nL, nS=2}
      mask prompts: nL "Link Number"; nS "Sensor ID of that link"
      mask DialogControl DescGroupVar Prompt: Virtual IMU
      mask DialogControl DescTextVar Prompt: Measures Connected Body's acceleration and angular velocity in the given point
      mask DialogControl Control2 Prompt: The following numbers defines the corresponding numbers for this sensor to read from the parameters file
  Terminator{,1..3} (4 alike) : Terminator
  Body Coord : PMIOPort  Port=1  Side=Left
  Reference Coord : PMIOPort  Port=2  Side=Left
  Out1 : Outport
  Out2 : Outport  Port=2
  Out5 : Outport  Port=3
  Out6 : Outport  Port=4
  wires:
  Sensor Module2/3(Out2) -> Terminator2/1
  Sensor Module2/1(Out5) -> Out5/1
  Sensor Module2/4(Out3) -> Terminator3/1
  Sensor Module2/2(Out4) -> Out6/1
  Sensor Module1/1(Out5) -> Out1/1
  Sensor Module1/4(Out3) -> Terminator1/1
  Sensor Module1/2(Out4) -> Out2/1
  Sensor Module1/3(Out2) -> Terminator/1
  connections:
  Sensor Module1/LConn1 -- Body Coord/RConn1 -- Sensor Module2/LConn1
  Sensor Module1/LConn2 -- Reference Coord/RConn1 -- Sensor Module2/LConn2

== system AariaJoystickR2017a/Joint4/JointVSS/PrismaticMotion/IMU Sensors ==
  Sensor Module1 : Subsystem  mask{nL=nL, nS=1}
      mask prompts: nL "Link Number"; nS "Sensor ID of that link"
      mask DialogControl DescGroupVar Prompt: Virtual IMU
      mask DialogControl DescTextVar Prompt: Measures Connected Body's acceleration and angular velocity in the given point
      mask DialogControl Control2 Prompt: The following numbers defines the corresponding numbers for this sensor to read from the parameters file
  Sensor Module2 : Subsystem  mask{nL=nL, nS=2}
      mask prompts: nL "Link Number"; nS "Sensor ID of that link"
      mask DialogControl DescGroupVar Prompt: Virtual IMU
      mask DialogControl DescTextVar Prompt: Measures Connected Body's acceleration and angular velocity in the given point
      mask DialogControl Control2 Prompt: The following numbers defines the corresponding numbers for this sensor to read from the parameters file
  Terminator{,1..3} (4 alike) : Terminator
  Body Coord : PMIOPort  Port=1  Side=Left
  Reference Coord : PMIOPort  Port=2  Side=Left
  Out1 : Outport
  Out2 : Outport  Port=2
  Out5 : Outport  Port=3
  Out6 : Outport  Port=4
  wires:
  Sensor Module1/3(Out2) -> Terminator/1
  Sensor Module1/2(Out4) -> Out2/1
  Sensor Module1/4(Out3) -> Terminator1/1
  Sensor Module1/1(Out5) -> Out1/1
  Sensor Module2/2(Out4) -> Out6/1
  Sensor Module2/4(Out3) -> Terminator3/1
  Sensor Module2/1(Out5) -> Out5/1
  Sensor Module2/3(Out2) -> Terminator2/1
  connections:
  Sensor Module2/LConn2 -- Reference Coord/RConn1 -- Sensor Module1/LConn2
  Sensor Module2/LConn1 -- Body Coord/RConn1 -- Sensor Module1/LConn1

== system AariaJoystickR2017a/Joint4/JointVSS/PrismaticMotion/x 2motion ==
  X : Inport
  Difference : simulink/Discrete/Difference  ICPrevInput=1  InputProcessing=Inherited  OutMin=[]  OutMax=[]  OutDataType=fixdt(1, 16)  OutScaling=2^-10  DoSatur=off
  Difference1 : simulink/Discrete/Difference  ICPrevInput=0  InputProcessing=Inherited  OutMin=[]  OutMax=[]  OutDataType=fixdt(1, 16)  OutScaling=2^-10  DoSatur=off
  Simulink-PS Converter : nesl_utility/Simulink-PS Converter  PhysicalDomain=network_engine_domain  SubClassName=ps_input  LeftPortType=input  RightPortType=output  PseudoPeriodic=off  Frequencies=[]  NoiseDistribution=none  NoiseParameters=[]  Unit=1  AffineConversion=off  FilteringAndDerivatives=provide  SimscapeFilterOrder=1  InputFilterTimeConstant=0.001  UdotUserProvided=2
  Motion for PS : PMIOPort  Port=1  Side=Right
  wires:
  Difference1/1 -> Simulink-PS Converter/2, Difference/1
  Difference/1 -> Simulink-PS Converter/3
  X/1 -> Difference1/1, Simulink-PS Converter/1
  connections:
  Simulink-PS Converter/RConn1 -- Motion for PS/RConn1

== system AariaJoystickR2017a/Joint4/JointVSS/PrismaticTorque/IMU Sensors ==
  Sensor Module1 : Subsystem  mask{nL=nL, nS=1}
      mask prompts: nL "Link Number"; nS "Sensor ID of that link"
      mask DialogControl DescGroupVar Prompt: Virtual IMU
      mask DialogControl DescTextVar Prompt: Measures Connected Body's acceleration and angular velocity in the given point
      mask DialogControl Control2 Prompt: The following numbers defines the corresponding numbers for this sensor to read from the parameters file
  Sensor Module2 : Subsystem  mask{nL=nL, nS=2}
      mask prompts: nL "Link Number"; nS "Sensor ID of that link"
      mask DialogControl DescGroupVar Prompt: Virtual IMU
      mask DialogControl DescTextVar Prompt: Measures Connected Body's acceleration and angular velocity in the given point
      mask DialogControl Control2 Prompt: The following numbers defines the corresponding numbers for this sensor to read from the parameters file
  Terminator{,1..3} (4 alike) : Terminator
  Body Coord : PMIOPort  Port=1  Side=Left
  Reference Coord : PMIOPort  Port=2  Side=Left
  Out1 : Outport
  Out2 : Outport  Port=2
  Out5 : Outport  Port=3
  Out6 : Outport  Port=4
  wires:
  Sensor Module1/3(Out2) -> Terminator/1
  Sensor Module1/2(Out4) -> Out2/1
  Sensor Module1/4(Out3) -> Terminator1/1
  Sensor Module1/1(Out5) -> Out1/1
  Sensor Module2/2(Out4) -> Out6/1
  Sensor Module2/4(Out3) -> Terminator3/1
  Sensor Module2/1(Out5) -> Out5/1
  Sensor Module2/3(Out2) -> Terminator2/1
  connections:
  Sensor Module2/LConn2 -- Reference Coord/RConn1 -- Sensor Module1/LConn2
  Sensor Module2/LConn1 -- Body Coord/RConn1 -- Sensor Module1/LConn1

== system AariaJoystickR2017a/Joint4/JointVSS/RevoluteMotion/IMU Sensors ==
  Sensor Module1 : Subsystem  mask{nL=nL, nS=1}
      mask prompts: nL "Link Number"; nS "Sensor ID of that link"
      mask DialogControl DescGroupVar Prompt: Virtual IMU
      mask DialogControl DescTextVar Prompt: Measures Connected Body's acceleration and angular velocity in the given point
      mask DialogControl Control2 Prompt: The following numbers defines the corresponding numbers for this sensor to read from the parameters file
  Sensor Module2 : Subsystem  mask{nL=nL, nS=2}
      mask prompts: nL "Link Number"; nS "Sensor ID of that link"
      mask DialogControl DescGroupVar Prompt: Virtual IMU
      mask DialogControl DescTextVar Prompt: Measures Connected Body's acceleration and angular velocity in the given point
      mask DialogControl Control2 Prompt: The following numbers defines the corresponding numbers for this sensor to read from the parameters file
  Terminator{,1..3} (4 alike) : Terminator
  Body Coord : PMIOPort  Port=1  Side=Left
  Reference Coord : PMIOPort  Port=2  Side=Left
  Out1 : Outport
  Out2 : Outport  Port=2
  Out5 : Outport  Port=3
  Out6 : Outport  Port=4
  wires:
  Sensor Module1/3(Out2) -> Terminator/1
  Sensor Module1/2(Out4) -> Out2/1
  Sensor Module1/4(Out3) -> Terminator1/1
  Sensor Module1/1(Out5) -> Out1/1
  Sensor Module2/2(Out4) -> Out6/1
  Sensor Module2/4(Out3) -> Terminator3/1
  Sensor Module2/1(Out5) -> Out5/1
  Sensor Module2/3(Out2) -> Terminator2/1
  connections:
  Sensor Module2/LConn2 -- Reference Coord/RConn1 -- Sensor Module1/LConn2
  Sensor Module2/LConn1 -- Body Coord/RConn1 -- Sensor Module1/LConn1
